simulink library "FE11_Batteries_lib"  (R2024a)
settings: Solver=VariableStepAuto  StartTime=0.0  StopTime=10.0  RelTol=1e-3
(part 1 of 2)
settings Model: Creator=laptop  LastModifiedBy=laptop

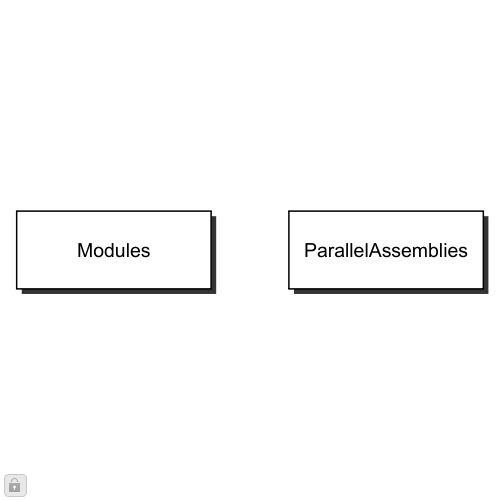
[thumbnail: Simulink's stored preview of the top-level diagram]
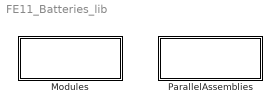
== system FE11_Batteries_lib ==
  Modules : Subsystem  Tag=simscape_sublibrary
      mask Display: disp(get_param(gcb,'Name'))
  ParallelAssemblies : Subsystem  Tag=simscape_sublibrary
      mask Display: disp(get_param(gcb,'Name'))

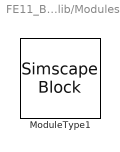
== system FE11_Batteries_lib/Modules ==
  ModuleType1 : SimscapeBlock  DialogController=NetworkEngine.DynNeDlgSource  LoadFcn=|  SourceFile=Batteries.Modules.ModuleType1  mask(ModuleType1){ComponentPath=Batteries.Modules.ModuleType1, ComponentVariants=["Batteries.Modules.ModuleType1"], ComponentVariantNames=["ModuleType1"], ClassName=ModuleType1, SchemaVersion=1, SOC_vecCell=[0, .01, .02, .03, .04, .05, .06, .07, .08, .09, .1, .11, .12, .13, .14, .15, .16, .17, .18, .19, .2, .21, .22, .23, .24, .25, .26, .27, .28, .29, .3, .31, .32, .33, .34, .35, .36, .37, .38, .39, .4, .41, .42, .43, .44, .45, .46, .47, .48, .49, .5, .51, .52, .53, .54, .55, .56, .57, .58, .59, .6, .61, .62, .63, .64, .65, .66, .67, .68, .69, .7, .71, .72, .73, .74, .75, .76, .77, .78, .79, .8, .81, .82, .83, .84, .85, .86, .87, .88, .89, .9, .91, .92, .93, .94, .95, .96, .97, .98, .99, 1], SOC_vecCell_unit=1, SOC_vecCell_conf=compiletime, T_vecCell=[-40, -30, -20, 0, 23, 45, 60], T_vecCell_unit=degC, T_vecCell_conf=compiletime, V0_matCell=[3.17242, 3.17242, 3.17242, 3.17242, 3.17242, 3.17242, 3.17242; 3.18272, 3.18272, 3.18272, 3.18272, 3.18272, 3.18272, 3.18272; 3.19302, 3.19302, 3.19302, 3.19302, 3.19302, 3.19302, 3.19302; 3.20331, 3.20331, 3.20331, 3.20331, 3.20331, 3.20331, 3.20331; 3.21361, 3.21361, 3.21361, 3.21361, 3.21361, 3.21361, 3.21361; 3.22391, 3.22391, 3.22391, 3.22391, 3.22391, 3.22391, 3.22391; 3.23421, 3.23421, 3.23421, 3.23421, 3.23421, 3.23421, 3.23421; 3.24451, 3.24451, 3.24451, 3.24451, 3.24451, 3.24451, 3.24451; 3.25481, 3.25481, 3.25481, 3.25481, 3.25481, 3.25481, 3.25481; 3.2651, 3.2651, 3.2651, 3.2651, 3.2651, 3.2651, 3.2651; 3.2754, 3.2754, 3.2754, 3.2754, 3.2754, 3.2754, 3.2754; 3.2857, 3.2857, 3.2857, 3.2857, 3.2857, 3.2857, 3.2857; 3.296, 3.296, 3.296, 3.296, 3.296, 3.296, 3.296; 3.3063, 3.3063, 3.3063, 3.3063, 3.3063, 3.3063, 3.3063; 3.31659, 3.31659, 3.31659, 3.31659, 3.31659, 3.31659, 3.31659; 3.32689, 3.32689, 3.32689, 3.32689, 3.32689, 3.32689, 3.32689; 3.33719, 3.33719, 3.33719, 3.33719, 3.33719, 3.33719, 3.33719; 3.34749, 3.34749, 3.34749, 3.34749, 3.34749, 3.34749, 3.34749; 3.35779, 3.35779, 3.35779, 3.35779, 3.35779, 3.35779, 3.35779; 3.36809, 3.36809, 3.36809, 3.36809, 3.36809, 3.36809, 3.36809; 3.37838, 3.37838, 3.37838, 3.37838, 3.37838, 3.37838, 3.37838; 3.38868, 3.38868, 3.38868, 3.38868, 3.38868, 3.38868, 3.38868; 3.39898, 3.39898, 3.39898, 3.39898, 3.39898, 3.39898, 3.39898; 3.40928, 3.40928, 3.40928, 3.40928, 3.40928, 3.40928, 3.40928; 3.41958, 3.41958, 3.41958, 3.41958, 3.41958, 3.41958, 3.41958; 3.42988, 3.42988, 3.42988, 3.42988, 3.42988, 3.42988, 3.42988; 3.44017, 3.44017, 3.44017, 3.44017, 3.44017, 3.44017, 3.44017; 3.45047, 3.45047, 3.45047, 3.45047, 3.45047, 3.45047, 3.45047; 3.46077, 3.46077, 3.46077, 3.46077, 3.46077, 3.46077, 3.46077; 3.47107, 3.47107, 3.47107, 3.47107, 3.47107, 3.47107, 3.47107; 3.48137, 3.48137, 3.48137, 3.48137, 3.48137, 3.48137, 3.48137; 3.49166, 3.49166, 3.49166, 3.49166, 3.49166, 3.49166, 3.49166; 3.50196, 3.50196, 3.50196, 3.50196, 3.50196, 3.50196, 3.50196; 3.51226, 3.51226, 3.51226, 3.51226, 3.51226, 3.51226, 3.51226; 3.52256, 3.52256, 3.52256, 3.52256, 3.52256, 3.52256, 3.52256; 3.53286, 3.53286, 3.53286, 3.53286, 3.53286, 3.53286, 3.53286; 3.54316, 3.54316, 3.54316, 3.54316, 3.54316, 3.54316, 3.54316; 3.55345, 3.55345, 3.55345, 3.55345, 3.55345, 3.55345, 3.55345; 3.56375, 3.56375, 3.56375, 3.56375, 3.56375, 3.56375, 3.56375; 3.57405, 3.57405, 3.57405, 3.57405, 3.57405, 3.57405, 3.57405; 3.58435, 3.58435, 3.58435, 3.58435, 3.58435, 3.58435, 3.58435; 3.59465, 3.59465, 3.59465, 3.59465, 3.59465, 3.59465, 3.59465; 3.60495, 3.60495, 3.60495, 3.60495, 3.60495, 3.60495, 3.60495; 3.61524, 3.61524, 3.61524, 3.61524, 3.61524, 3.61524, 3.61524; 3.62554, 3.62554, 3.62554, 3.62554, 3.62554, 3.62554, 3.62554; 3.63584, 3.63584, 3.63584, 3.63584, 3.63584, 3.63584, 3.63584; 3.64614, 3.64614, 3.64614, 3.64614, 3.64614, 3.64614, 3.64614; 3.65644, 3.65644, 3.65644, 3.65644, 3.65644, 3.65644, 3.65644; 3.66673, 3.66673, 3.66673, 3.66673, 3.66673, 3.66673, 3.66673; 3.67703, 3.67703, 3.67703, 3.67703, 3.67703, 3.67703, 3.67703; 3.68733, 3.68733, 3.68733, 3.68733, 3.68733, 3.68733, 3.68733; 3.69763, 3.69763, 3.69763, 3.69763, 3.69763, 3.69763, 3.69763; 3.71041, 3.71041, 3.71041, 3.71041, 3.71041, 3.71041, 3.71041; 3.72113, 3.72113, 3.72113, 3.72113, 3.72113, 3.72113, 3.72113; 3.72997, 3.72997, 3.72997, 3.72997, 3.72997, 3.72997, 3.72997; 3.73882, 3.73882, 3.73882, 3.73882, 3.73882, 3.73882, 3.73882; 3.74912, 3.74912, 3.74912, 3.74912, 3.74912, 3.74912, 3.74912; 3.75936, 3.75936, 3.75936, 3.75936, 3.75936, 3.75936, 3.75936; 3.76951, 3.76951, 3.76951, 3.76951, 3.76951, 3.76951, 3.76951; 3.7791, 3.7791, 3.7791, 3.7791, 3.7791, 3.7791, 3.7791; 3.78865, 3.78865, 3.78865, 3.78865, 3.78865, 3.78865, 3.78865; 3.79787, 3.79787, 3.79787, 3.79787, 3.79787, 3.79787, 3.79787; 3.80709, 3.80709, 3.80709, 3.80709, 3.80709, 3.80709, 3.80709; 3.8161, 3.8161, 3.8161, 3.8161, 3.8161, 3.8161, 3.8161; 3.82509, 3.82509, ...(+2298 chars)], V0_matCell_unit=V, V0_matCell_conf=compiletime, V_rangeCell=[2.25, Inf], V_rangeCell_unit=V, V_rangeCell_conf=compiletime, R0_matCell=[.3026, .35142, .34349, .24415, .02095, .15874, .14729; .2941, .33555, .32379, .22614, .01921, .13363, .12249; .28559, .31969, .30408, .20813, .01774, .10853, .10276; .27709, .30382, .28438, .19012, .0166, .09423, .0861; .26858, .28796, .26468, .17211, .01557, .07998, .0748; .26008, .27209, .24498, .1541, .01469, .07024, .06679; .25157, .25623, .22527, .1361, .01398, .06387, .05877; .24307, .24036, .20557, .11861, .01338, .0575, .05275; .23456, .2245, .18587, .10674, .01283, .05113, .04899; .22606, .20863, .16617, .09525, .01239, .04679, .04522; .21755, .19277, .14651, .08799, .01196, .0439, .04145; .20905, .1769, .13098, .08073, .01155, .04101, .03817; .20054, .16103, .11905, .07347, .01116, .03813, .03522; .19204, .14769, .11102, .06895, .01079, .03524, .03228; .18353, .13913, .10517, .06499, .01042, .03235, .02934; .17503, .13157, .09933, .06104, .01007, .02946, .0264; .16653, .1271, .09371, .05708, .00974, .02657, .02345; .15804, .12264, .09094, .05312, .00949, .02417, .02125; .15354, .11817, .08816, .04917, .00924, .02286, .01972; .14976, .11385, .08539, .04748, .009, .02156, .0182; .14598, .11213, .08261, .04617, .00876, .02025, .01667; .14219, .11042, .08103, .04487, .00855, .01894, .01515; .14033, .10871, .08035, .04356, .00843, .01763, .01363; .13876, .10699, .07967, .04225, .00832, .01632, .0121; .13718, .10528, .07899, .04094, .00826, .01501, .01058; .13561, .10357, .07831, .03964, .00825, .0137, .00906; .13404, .10198, .07763, .03833, .00825, .01239, .00753; .13247, .10119, .07695, .03702, .00826, .01108, .0065; .13096, .10039, .07627, .03624, .00827, .00977, .00633; .13043, .0996, .07559, .03615, .00828, .00846, .00617; .1299, .0988, .07491, .03606, .0083, .00774, .006; .12937, .09801, .07423, .03597, .00834, .00779, .00583; .12883, .09721, .07355, .03588, .00838, .00783, .00567; .1283, .09642, .07301, .03579, .00842, .00787, .0055; .12777, .09585, .07296, .0357, .00848, .00792, .00534; .12724, .09584, .07291, .03561, .00855, .00796, .00517; .12675, .09584, .07286, .03552, .00863, .00801, .005; .12643, .09583, .0728, .03543, .00871, .00805, .00484; .12611, .09582, .07275, .03534, .00879, .00809, .00467; .12579, .09582, .0727, .03525, .00887, .00814, .0045; .12547, .09581, .07264, .03526, .00895, .00818, .00434; .12514, .0958, .07259, .03537, .00903, .00823, .00405; .12482, .09579, .07254, .03547, .00911, .00804, .00366; .1245, .09579, .07248, .03558, .00918, .00776, .00327; .12418, .09578, .07243, .03568, .00925, .00748, .00287; .12386, .09577, .07231, .03579, .00931, .0072, .00248; .12354, .09576, .0721, .03589, .00938, .00692, .00209; .12322, .09576, .07189, .036, .00946, .00664, .0017; .12301, .09575, .07168, .03611, .00953, .00636, .00131; .12309, .09574, .07147, .03621, .00961, .00608, .00092; .12318, .09573, .07125, .0363, .00968, .0058, .00053; .12326, .09573, .07104, .03637, .00976, .00552, .00014; .12389, .09628, .07138, .03699, .00991, .00579, .0003; .12407, .09637, .07126, .03715, .01, .0056, .0003; .12383, .09605, .07073, .0369, .01003, .00504, .0003; .12359, .09573, .07019, .03664, .01006, .00503, .0003; .12367, .09573, .06998, .03671, .01013, .00534, .00063; .12375, .09572, .06975, .03677, .01022, .00564, .00094; .1238, .09569, .07006, .0368, .0103, .00593, .00123; .12372, .09554, .07026, .03671, .01037, .00608, .00139; .12364, .09537, .07046, .03661, .01043, .00623, .00155; .12348, .09514, .07058, .03644, .01049, .0063, .00163; .12333, .0949, .07071, .03627, .01055, .00638, .00171; .12312, .09461, .07078, .03605, .01061, .00641, .00175; .12291, .09433, .07085, .03583, .01066, .00643, .00168; .12271, .09404, .07093, .03568, .01072, .00646, .00161; .12275, .09398, .071, .03622, .01077, .00646, .00153; .12316, .09449, .07107, .03677, .01082, .00636, .00145; .12357, .095, .07115, .03731, .01088, .00625, .00137; .12398, .09551, .07151, .03785, .01093, .00614, .00129; .12438, .09601, .07221, .03839, .01099, .00602, .0012; .12486, .09659, .07299, .039, .01105, .00599, .00119; .12548, .09731, .07391, ...(+1578 chars)], R0_matCell_unit=Ohm, R0_matCell_conf=compiletime, AHCell=4.493, AHCell_unit=A*hr, AHCell_conf=compiletime, extrapolation_optionCell=simscape.enum.extrapolation.nearest, extrapolation_optionCell_unit=1, extrapolation_optionCell_conf=compiletime, thermal_massCell=63, thermal_massCell_unit=J/K, thermal_massCell_conf=compiletime, AmbientResistance=25, AmbientResistance_unit=K/W, AmbientResistance_conf=compiletime, CellBalancingClosedResistance=0.01, CellBalancingClosedResistance_unit=Ohm, CellBalancingClosedResistance_conf=compiletime, CellBalancingOpenConductance=1e-8, CellBalancingOpenConductance_unit=1/Ohm, CellBalancingOpenConductance_conf=compiletime, CellBalancingThreshold=0.5, CellBalancingThreshold_unit=1, CellBalancingThreshold_conf=compiletime, CellBalancingResistance=50, CellBalancingResistance_unit=Ohm, CellBalancingResistance_conf=compiletime, P=4, P_unit=1, P_conf=compiletime, S=12, S_unit=1, S_conf=compiletime, iCell_specify=off, iCell_priority=None, iCell=0, iCell_unit=A, iCell_nominal_specify=off, iCell_nominal_value=1, iCell_nominal_unit=A, vCell_specify=off, vCell_priority=None, vCell=0, vCell_unit=V, vCell_nominal_specify=off, vCell_nominal_value=1, vCell_nominal_unit=V, socCell_specify=off, socCell_priority=High, socCell=1, socCell_unit=1, socCell_nominal_specify=off, socCell_nominal_value=1, socCell_nominal_unit=1, numCyclesCell_specify=off, numCyclesCell_priority=High, numCyclesCell=0, numCyclesCell_unit=1, numCyclesCell_nominal_specify=off, numCyclesCell_nominal_value=1, numCyclesCell_nominal_unit=1, temperatureCell_specify=off, temperatureCell_priority=High, temperatureCell=298.15, temperatureCell_unit=K, temperatureCell_nominal_specify=off, temperatureCell_nominal_value=1, temperatureCell_nominal_unit=K, vParallelAssembly_specify=off, vParallelAssembly_priority=None, vParallelAssembly=repmat(0, 12, 1), vParallelAssembly_unit=V, vParallelAssembly_nominal_specify=off, vParallelAssembly_nominal_value=1, vParallelAssembly_nominal_unit=V, socParallelAssembly_specify=off, socParallelAssembly_priority=None, socParallelAssembly=repmat(1, 12, 1), socParallelAssembly_unit=1, socParallelAssembly_nominal_specify=off, socParallelAssembly_nominal_value=1, socParallelAssembly_nominal_unit=1}
      | simscape.compiler.sli.internal.callback('LoadFcn',gcbh);
      | battery_builder_rtmsupport('loadfcn',gcbh);
      mask prompts: SOC_vecCell "Vector of state-of-charge values, SOC"; T_vecCell "Vector of temperatures, T"; V0_matCell "Open-circuit voltage, V0(SOC,T)"; V_rangeCell "Terminal voltage operating range [Min Max]"; R0_matCell "Terminal resistance, R0(SOC,T)"; AHCell "Cell capacity, AH"; extrapolation_optionCell "Extrapolation method for all tables"; thermal_massCell "Thermal mass"; AmbientResistance "Cell level ambient thermal path resistance"; CellBalancingClosedResistance "Cell balancing switch closed resistance"; CellBalancingOpenConductance "Cell balancing switch open conductance"; CellBalancingThreshold "Cell balancing switch operation threshold"; CellBalancingResistance "Cell balancing shunt resistance"; P "Batteries in Parallel"; S "Batteries in Series"; iCell_specify "Cell current (positive in)"; iCell_priority "physmod:common:pi:sli:kernel:VariablePriority"; iCell "physmod:common:pi:sli:kernel:VariableValue"; iCell_nominal_specify "Cell current (positive in)"; iCell_nominal_value "physmod:common:pi:sli:kernel:VariableValue"; vCell_specify "Cell terminal voltage"; vCell_priority "physmod:common:pi:sli:kernel:VariablePriority"; vCell "physmod:common:pi:sli:kernel:VariableValue"; vCell_nominal_specify "Cell terminal voltage"; vCell_nominal_value "physmod:common:pi:sli:kernel:VariableValue"; socCell_specify "Cell state of charge"; socCell_priority "physmod:common:pi:sli:kernel:VariablePriority"; socCell "physmod:common:pi:sli:kernel:VariableValue"; socCell_nominal_specify "Cell state of charge"; socCell_nominal_value "physmod:common:pi:sli:kernel:VariableValue"; numCyclesCell_specify "Cell discharge cycles"; numCyclesCell_priority "physmod:common:pi:sli:kernel:VariablePriority"; numCyclesCell "physmod:common:pi:sli:kernel:VariableValue"; numCyclesCell_nominal_specify "Cell discharge cycles"; numCyclesCell_nominal_value "physmod:common:pi:sli:kernel:VariableValue"; temperatureCell_specify "Cell temperature"; temperatureCell_priority "physmod:common:pi:sli:kernel:VariablePriority"; temperatureCell "physmod:common:pi:sli:kernel:VariableValue"; temperatureCell_nominal_specify "Cell temperature"; temperatureCell_nominal_value "physmod:common:pi:sli:kernel:VariableValue"; vParallelAssembly_specify "Parallel Assembly Voltage"; vParallelAssembly_priority "physmod:common:pi:sli:kernel:VariablePriority"; vParallelAssembly "physmod:common:pi:sli:kernel:VariableValue"; vParallelAssembly_nominal_specify "Parallel Assembly Voltage"; vParallelAssembly_nominal_value "physmod:common:pi:sli:kernel:VariableValue"; socParallelAssembly_specify "Parallel Assembly state of charge"; socParallelAssembly_priority "physmod:common:pi:sli:kernel:VariablePriority"; socParallelAssembly "physmod:common:pi:sli:kernel:VariableValue"; socParallelAssembly_nominal_specify "Parallel Assembly state of charge"; socParallelAssembly_nominal_value "physmod:common:pi:sli:kernel:VariableValue"
      mask help:
      | Module Block
      |    Model resolution: Lumped
      |    Number of parallel assemblies: 12
      |    Number of cells per parallel assembly: 4
      |
      | Block is parameterized for this Battery:
      |    Part number: INR_21700_P45B
      |    Manufacturer: Molicel
      |    Web link: https://www.molicel.com/
      |    Parameterization note: Predefined parameterizations of Simscape components use available data sources for supplying parameter values. Engineering judgement and simplifying assumptions are used to fill in for missing data. As a result, deviations between simulated and actual physical behavior should be expected. To ensure requisite accuracy, you should validate simulated behavior against experimental data and refine component models as necessary.
      |
      |    MATLAB version: 24.1
      |    Simscape Battery version: 24.1
      |    Simscape code generated on: 05-Aug-2024 18:24:07
      mask init:
      | simscape.compiler.sli.internal.preinitmask(gcb);
      settings: DeleteFcn=simscape.compiler.sli.internal.callback('DeleteFcn',gcbh);  ModelCloseFcn=simscape.compiler.sli.internal.callback('ModelCloseFcn',gcbh);  PreSaveFcn=simscape.compiler.sli.internal.callback('PreSaveFcn',gcbh);  PostSaveFcn=simscape.compiler.sli.internal.callback('PostSaveFcn',gcbh);  InternalSimscapePortConfiguration="{\"Bottom\":[{\"id\":\"n\",\"label\":\"-\",\"type\":\"foundation.electrical.electrical\"}],\"Left\":[{\"id\":\"enableCellBalancing\",\"label\":\"CB\",\"type\":\"input\"},{\"id\":\"AmbH\",\"label\":\"AmbH\",\"type\":\"foundation.thermal.thermal\"}],\"Right\":[],\"Top\":[{\"id\":\"p\",\"label\":\"+\",\"type\":\"foundation.electrical.electrical\"}]}"
      settings: CopyFcn=|
      | simscape.compiler.sli.internal.callback('CopyFcn',gcbh);
      | battery_builder_rtmsupport('copyfcn',gcbh);
      settings: PreCopyFcn=|
      | simscape.compiler.sli.internal.callback('PreCopyFcn',gcbh);
      | battery_builder_rtmsupport('precopyfcn',gcbh);
      settings: PreDeleteFcn=|
      | simscape.compiler.sli.internal.callback('PreDeleteFcn',gcbh);
      | battery_builder_rtmsupport('predeletefcn',gcbh);
      mask Help: web(nesl_help(gcbh))
      mask TypeOptions SOC_vecCell_unit: 1
      mask TypeOptions SOC_vecCell_conf: compiletime | runtime
      mask TypeOptions T_vecCell_unit: K | degC | degF | degR | deltaK | deltadegC | deltadegF | deltadegR
      mask TypeOptions T_vecCell_conf: compiletime | runtime
      mask TypeOptions V0_matCell_unit: V | MV | kV | mV
      mask TypeOptions V0_matCell_conf: compiletime | runtime
      mask TypeOptions V_rangeCell_unit: V | MV | kV | mV
      mask TypeOptions V_rangeCell_conf: compiletime | runtime
      mask TypeOptions R0_matCell_unit: Ohm | GOhm | MOhm | kOhm | mOhm
      mask TypeOptions R0_matCell_conf: compiletime | runtime
      mask TypeOptions AHCell_unit: C | Ah | mC | nC | uC | MAh | kAh | mAh | A*hr
      mask TypeOptions AHCell_conf: compiletime | runtime
      mask TypeOptions extrapolation_optionCell: simscape.enum.extrapolation.linear | simscape.enum.extrapolation.nearest | simscape.enum.extrapolation.error
      mask TypeOptions extrapolation_optionCell_unit: 1
      mask TypeOptions extrapolation_optionCell_conf: compiletime
      mask TypeOptions thermal_massCell_unit: J/K
      mask TypeOptions thermal_massCell_conf: compiletime | runtime
      mask TypeOptions AmbientResistance_unit: K/W
      mask TypeOptions AmbientResistance_conf: compiletime | runtime
      mask TypeOptions CellBalancingClosedResistance_unit: Ohm | GOhm | MOhm | kOhm | mOhm
      mask TypeOptions CellBalancingClosedResistance_conf: compiletime | runtime
      mask TypeOptions CellBalancingOpenConductance_unit: S | mS | nS | uS | 1/Ohm
      mask TypeOptions CellBalancingOpenConductance_conf: compiletime | runtime
      mask TypeOptions CellBalancingThreshold_unit: 1
      mask TypeOptions CellBalancingThreshold_conf: compiletime | runtime
      mask TypeOptions CellBalancingResistance_unit: Ohm | GOhm | MOhm | kOhm | mOhm
      mask TypeOptions CellBalancingResistance_conf: compiletime | runtime
      mask TypeOptions P_unit: 1
      mask TypeOptions P_conf: compiletime | runtime
      mask TypeOptions S_unit: 1
      mask TypeOptions S_conf: compiletime
      mask TypeOptions iCell_priority: None | Low | High
      mask TypeOptions iCell_unit: A | MA | kA | mA | nA | pA | uA
      mask TypeOptions iCell_nominal_unit: A | MA | kA | mA | nA | pA | uA
      mask TypeOptions vCell_priority: None | Low | High
      mask TypeOptions vCell_unit: V | MV | kV | mV
      mask TypeOptions vCell_nominal_unit: V | MV | kV | mV
      mask TypeOptions socCell_priority: None | Low | High
      mask TypeOptions socCell_unit: 1
      mask TypeOptions socCell_nominal_unit: 1
      mask TypeOptions numCyclesCell_priority: None | Low | High
      mask TypeOptions numCyclesCell_unit: 1
      mask TypeOptions numCyclesCell_nominal_unit: 1
      mask TypeOptions temperatureCell_priority: None | Low | High
      mask TypeOptions temperatureCell_unit: K | degC | degF | degR | deltaK | deltadegC | deltadegF | deltadegR
      mask TypeOptions temperatureCell_nominal_unit: K | degC | degF | degR | deltaK | deltadegC | deltadegF | deltadegR
      mask TypeOptions vParallelAssembly_priority: None | Low | High
      mask TypeOptions vParallelAssembly_unit: V | MV | kV | mV
      mask TypeOptions vParallelAssembly_nominal_unit: V | MV | kV | mV
      mask TypeOptions socParallelAssembly_priority: None | Low | High
      mask TypeOptions socParallelAssembly_unit: 1
      mask TypeOptions socParallelAssembly_nominal_unit: 1
      mask DialogControl simscape__settings__group__ Prompt: physmod:common:gui:mli:schema:PISettingsTab
      mask DialogControl simscape__internal__group__name__1 Prompt: Main
      mask DialogControl simscape__internal__group__name__2 Prompt: Thermal
      mask DialogControl simscape__internal__group__name__3 Prompt: Cell Balancing
      mask DialogControl simscape__internal__group__name__4 Prompt: Initial Targets
      mask DialogControl iCell_priority Prompt: Priority
      mask DialogControl iCell Prompt: Value
      mask DialogControl vCell_priority Prompt: Priority
      mask DialogControl vCell Prompt: Value
      mask DialogControl socCell_priority Prompt: Priority
      mask DialogControl socCell Prompt: Value
      mask DialogControl numCyclesCell_priority Prompt: Priority
      mask DialogControl numCyclesCell Prompt: Value
      mask DialogControl temperatureCell_priority Prompt: Priority
      mask DialogControl temperatureCell Prompt: Value
      mask DialogControl vParallelAssembly_priority Prompt: Priority
      mask DialogControl vParallelAssembly Prompt: Value
      mask DialogControl socParallelAssembly_priority Prompt: Priority
      mask DialogControl socParallelAssembly Prompt: Value
      mask DialogControl simscape__internal__group__name__5 Prompt: physmod:common:pi:sli:cs2ps:NominalContainer
      mask DialogControl iCell_nominal_value Prompt: Value
      mask DialogControl vCell_nominal_value Prompt: Value
      mask DialogControl socCell_nominal_value Prompt: Value
      mask DialogControl numCyclesCell_nominal_value Prompt: Value
      mask DialogControl temperatureCell_nominal_value Prompt: Value
      mask DialogControl vParallelAssembly_nominal_value Prompt: Value
      mask DialogControl socParallelAssembly_nominal_value Prompt: Value
